simulink model "one_heater"  (R2023b)
settings: Solver=FixedStepAuto  StartTime=0.0  StopTime=1200  FixedStep=1  RelTol=1e-3
values from neighbouring files (symbols this model uses):
  A = 7e-4    (= 0.0007)    [dual_heater1.m]    (also in one_heater1.m = 0.0012)
  alfa = 0.9    [dual_heater1.m]    (also in one_heater1.m = 0.5)
  C2K = 273.15    [dual_heater1.m]    (also in one_heater1.m)
  cp = 500    [dual_heater1.m]    (also in one_heater1.m)
  m = 4e-3    (= 0.004)    [dual_heater1.m]    (also in one_heater1.m)
  sig = 5.67e-8    (= 5.67e-08)    [dual_heater1.m]    (also in one_heater1.m)
  T = T + C2K    (= 296.15)    [dual_heater1.m]    (also in one_heater1.m)
  t0 = t0 + C2K    (= 296.15)    [dual_heater1.m]    (also in one_heater1.m)
  U = 10    [dual_heater1.m]    (also in one_heater1.m)
settings Model: Creator=ondre  LastModifiedBy=ondre

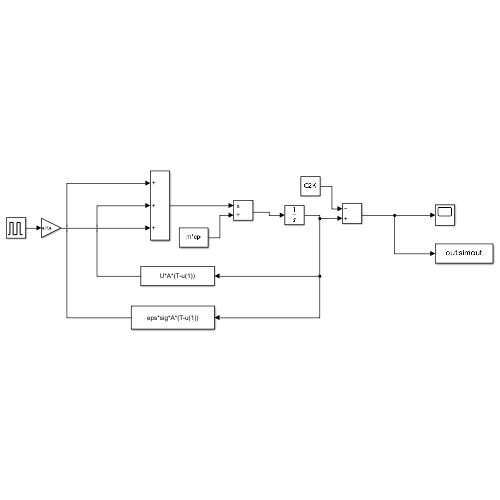
[thumbnail: Simulink's stored preview of the top-level diagram]
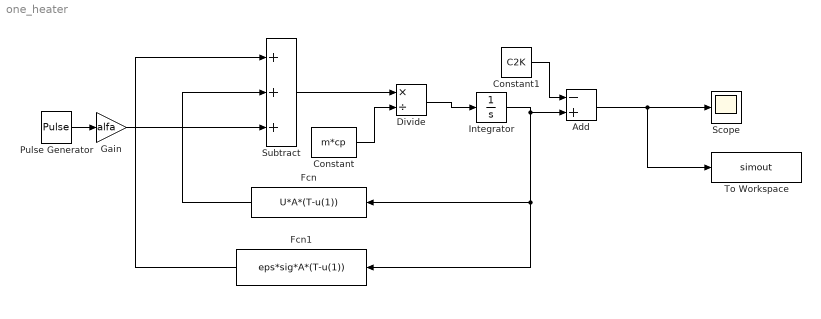
== system one_heater ==
  Add : Sum  Inputs=-+
  Constant : Constant  Value=m*cp
  Constant1 : Constant  Value=C2K
  Divide : Product  Inputs=*/
  Fcn : Fcn  Expr=U*A*(T-u(1))
  Fcn1 : Fcn  Expr=eps*sig*A*(T-u(1))
  Gain : Gain  Gain=alfa
  Integrator : Integrator  InitialCondition=t0
  Pulse Generator : DiscretePulseGenerator  PulseType=Time based  Period=1200  PulseWidth=50
  Scope : Scope
  Subtract : Sum  Inputs=+++
  To Workspace : ToWorkspace  VariableName=simout  SaveFormat=Structure With Time  SampleTime=-1
  wires:
  Subtract/1 -> Divide/1
  Divide/1 -> Integrator/1
  Constant/1 -> Divide/2
  Integrator/1 -> Add/2, Fcn1/1, Fcn/1
  Fcn/1 -> Subtract/2
  Fcn1/1 -> Subtract/1
  Pulse Generator/1 -> Gain/1
  Gain/1 -> Subtract/3
  Add/1 -> To Workspace/1, Scope/1
  Constant1/1 -> Add/1
